simulink model "lat_zengwen"  (R2016a)
settings: Solver=VariableStepAuto  StartTime=0.0  StopTime=200  RelTol=1e-3
undefined symbols (not defined in the file): Alat, Blat, Clat, Dlat
settings Model: Creator=Gray  LastModifiedBy=Gray

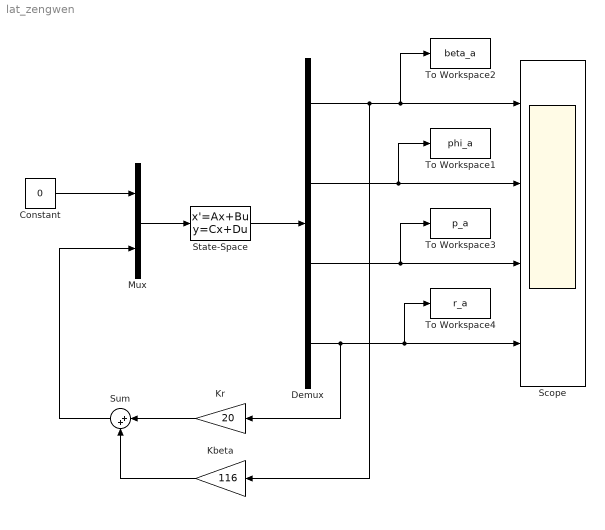
== system lat_zengwen ==
  Constant : Constant  Value=0
  Demux : Demux
  Kbeta : Gain  Gain=116
  Kr : Gain  Gain=20
  Mux : Mux  Inputs=2
  Scope : Scope  NumInputPorts=4
  State-Space : StateSpace  A=Alat  B=Blat  C=Clat  D=Dlat  X0="[5/57.3 0 0  0]'"
  Sum : Sum  Inputs=|++
  To Workspace1 : ToWorkspace  VariableName=phi_a  SaveFormat=Timeseries  SampleTime=-1
  To Workspace2 : ToWorkspace  VariableName=beta_a  SaveFormat=Timeseries  SampleTime=-1
  To Workspace3 : ToWorkspace  VariableName=p_a  SaveFormat=Timeseries  SampleTime=-1
  To Workspace4 : ToWorkspace  VariableName=r_a  SaveFormat=Timeseries  SampleTime=-1
  wires:
  State-Space/1 -> Demux/1
  Mux/1 -> State-Space/1
  Kbeta/1 -> Sum/2
  Kr/1 -> Sum/1
  Demux/2 -> To Workspace1/1, Scope/2
  Demux/4 -> Kr/1, To Workspace4/1, Scope/4
  Demux/1 -> Kbeta/1, To Workspace2/1, Scope/1
  Demux/3 -> To Workspace3/1, Scope/3
  Constant/1 -> Mux/1
  Sum/1 -> Mux/2
